simulink model "fig7_75"  (Simulink 8.4)
settings: Solver=ode45  StartTime=0.0  StopTime=100.0  RelTol=1e-3
libraries: simulink x1
settings Model: Creator=abbas  LastModifiedBy=abbas  ExtModeTrigMode=oneshot  ExtModeArmWhenConnect=off
settings DataIOCC: LimitDataPoints=off
settings OptimizationCC: BlockReduction=off  BooleanDataType=off  InitFltsAndDblsToZero=on
settings DebuggingCC: SaveWithParameterizedLinksMsg=none  SignalResolutionControl=TryResolveAllWithWarning  SolverPrmCheckMsg=none  MultiTaskDSMMsg=warning  MultiTaskCondExecSysMsg=none
settings HardwareCC: TargetUnknown=on
settings RTWCC: IncludeERTFirstTime=on
settings GRTTargetCC: TargetFcnLib=ansi_tfl_tmw.mat  ModelReferenceCompliant=off  ParMdlRefBuildCompliant=off  CompOptLevelCompliant=off  MatFileLogging=off

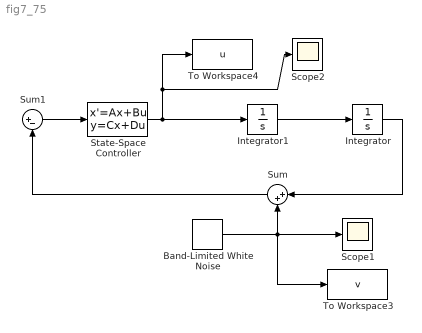
== system fig7_75 ==
  Band-Limited White Noise : simulink/Sources/Band-Limited White Noise  Cov=[0.1]  Ts=0.05  seed=[23341]
  Integrator : Integrator
  Integrator1 : Integrator
  Scope1 : Scope
      settings: YMin=-12.5  YMax=10
  Scope2 : Scope
      settings: YMin=-12.5  YMax=10
  State-Space Controller : StateSpace  A=[-14.1421 1;-101 -1.4142]  B=|  C="[1.0000    1.4142]"  D=[0]  X0=0
      | [14.1421;
      |   100.0000]
  Sum : Sum  Inputs=|++  SaturateOnIntegerOverflow=on  InputSameDT=on  OutDataTypeStr=Inherit: Same as first input
  Sum1 : Sum  Inputs=|+-  SaturateOnIntegerOverflow=on  InputSameDT=on  OutDataTypeStr=Inherit: Same as first input
  To Workspace3 : ToWorkspace  VariableName=v  SampleTime=0.0
  To Workspace4 : ToWorkspace  VariableName=u  SampleTime=0.0
  wires:
  Integrator1/1 -> Integrator/1
  Integrator/1 -> Sum/1
  Sum/1 -> Sum1/2
  Sum1/1 -> State-Space Controller/1
  Band-Limited White Noise/1 -> Sum/2, Scope1/1, To Workspace3/1
  State-Space Controller/1 -> Integrator1/1, To Workspace4/1, Scope2/1
